simulink model "Reaction_wheel_forse_earth_sensor"  (R2020b)
settings: Solver=VariableStepAuto  StartTime=0.0  StopTime=10.0  RelTol=1e-3
undefined symbols (not defined in the file or in its folder): A, A_star, B, J, Kt, Kw, lw, phi_max, rad, Rm, s, theta_max
libraries: aerolibconvert2 x2, simulink x2, pid_lib x1
settings Model: Creator=jason  LastModifiedBy=jason

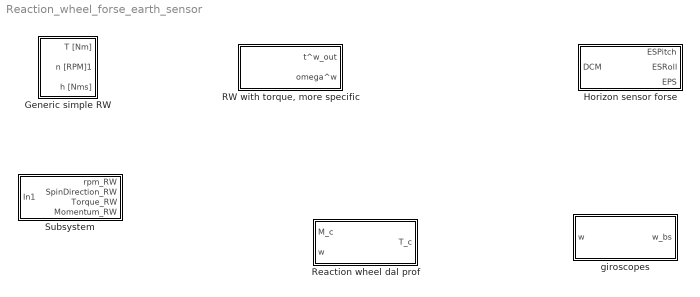
== system Reaction_wheel_forse_earth_sensor ==
  Generic simple RW : Subsystem
  Horizon sensor forse : Subsystem
  "RW with torque, more specific" : Subsystem
  Reaction wheel dal prof : Subsystem
  Subsystem : Subsystem
  giroscopes : Subsystem

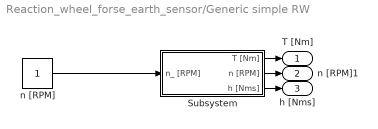
== system Reaction_wheel_forse_earth_sensor/Generic simple RW ==
  Subsystem : Subsystem
  n [RPM] : Constant
  T [Nm] : Outport
  n [RPM]1 : Outport  Port=2
  h [Nms] : Outport  Port=3
  wires:
  Subsystem/2(n [RPM]) -> n [RPM]1/1
  n [RPM]/1 -> Subsystem/1(n_ [RPM])
  Subsystem/1(T [Nm]) -> T [Nm]/1
  Subsystem/3(h [Nms]) -> h [Nms]/1

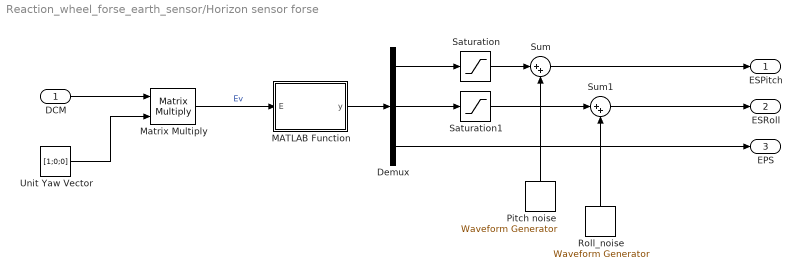
== system Reaction_wheel_forse_earth_sensor/Horizon sensor forse ==
  DCM : Inport
  Demux : Demux  Outputs=3
  MATLAB Function : MATLAB Function  TreatAsAtomicUnit=on
  Matrix Multiply : Product  Multiplication=Matrix(*)
  Pitch noise : simulink/Sources/Waveform Generator  OutMin=[]  OutMax=[]  OutDataTypeStr=double  SelectedSignal=1  BlockNames=MultiportSwitch_e3df3653d217406  SampleTime=0.1
  Roll_noise : simulink/Sources/Waveform Generator  OutMin=[]  OutMax=[]  OutDataTypeStr=double  SelectedSignal=1  BlockNames=MultiportSwitch_e3df3653d217406  SampleTime=0.1
  Saturation : Saturate  UpperLimit=theta_max  LowerLimit=-theta_max
  Saturation1 : Saturate  UpperLimit=phi_max  LowerLimit=-phi_max
  Sum : Sum  Inputs=|++
  Sum1 : Sum  Inputs=|++
  Unit Yaw Vector : Constant  Value=[1;0;0]
  ESPitch : Outport
  ESRoll : Outport  Port=2
  EPS : Outport  Port=3
  wires:
  DCM/1 -> Matrix Multiply/1
  Unit Yaw Vector/1 -> Matrix Multiply/2
  Matrix Multiply/1 -> MATLAB Function/1(E)  "Ev"
  MATLAB Function/1(y) -> Demux/1
  Demux/2 -> Saturation1/1
  Demux/1 -> Saturation/1
  Demux/3 -> EPS/1
  Saturation/1 -> Sum/1
  Saturation1/1 -> Sum1/1
  Sum1/1 -> ESRoll/1
  Sum/1 -> ESPitch/1
  Roll_noise/1 -> Sum1/2
  Pitch noise/1 -> Sum/2

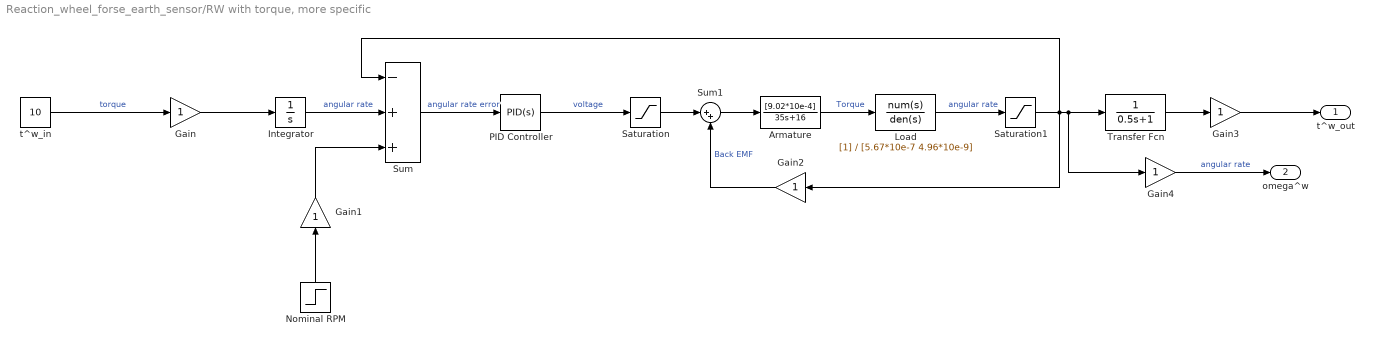
== system Reaction_wheel_forse_earth_sensor/RW with torque, more specific ==
  Armature : TransferFcn  Numerator=[9.02*10e-4]  Denominator=[35 16]  ContinuousStateAttributes='Armature'
  Gain{,1..4} (5 alike) : Gain
  Integrator : Integrator
  Load : TransferFcn  Denominator=[5.67*10e-7 4.96*10e-9]
  Nominal RPM : Step  Time=100  Before=18400  After=36800  SampleTime=0
  PID Controller : pid_lib/PID Controller  Controller=PID  Form=Parallel  TimeDomain=Continuous-time  UseExternalTs=off  SampleTime=-1  IntegratorMethod=Forward Euler  FilterMethod=Forward Euler  ControllerParametersSource=internal  P=9.7  I=0.666  D=0.4  UseFilter=on  N=100  TunerSelectOption=Transfer Function Based (PID Tuner App)  InitialConditionSource=internal  InitialConditionForIntegrator=0  InitialConditionForFilter=0  DifferentiatorICPrevScaledInput=0  ExternalReset=none  TrackingMode=off  Kt=1  LimitOutput=off  SatLimitsSource=internal  UpperSaturationLimit=inf  LowerSaturationLimit=-inf  LinearizeAsGain=on  AntiWindupMode=none  Kb=1  POutMin=[]  POutMax=[]  IOutMin=[]  IOutMax=[]  DOutMin=[]  DOutMax=[]  NOutMin=[]  NOutMax=[]  SumOutMin=[]  SumOutMax=[]  SaturationOutMin=[]  SaturationOutMax=[]  PParamMin=[]  PParamMax=[]  IParamMin=[]  IParamMax=[]  DParamMin=[]  DParamMax=[]  NParamMin=[]  NParamMax=[]  KbParamMin=[]  KbParamMax=[]  KtParamMin=[]  KtParamMax=[]  KbOutMin=[]  KbOutMax=[]  KtOutMin=[]  KtOutMax=[]  IntegratorOutMin=[]  IntegratorOutMax=[]  FilterOutMin=[]  FilterOutMax=[]  SumI1OutMin=[]  SumI1OutMax=[]  SumI2OutMin=[]  SumI2OutMax=[]  SumI3OutMin=[]  SumI3OutMax=[]  SumI4OutMin=[]  SumI4OutMax=[]  SumDOutMin=[]  SumDOutMax=[]  DifferentiatorOutMin=[]  DifferentiatorOutMax=[]  FilterDiffOutCoefMin=[]  FilterDiffOutCoefMax=[]  ReciprocalOutMin=[]  ReciprocalOutMax=[]  SumDenOutMin=[]  SumDenOutMax=[]  SumNumOutMin=[]  SumNumOutMax=[]  DivideOutMin=[]  DivideOutMax=[]  UdiffTsProdOutMin=[]  UdiffTsProdOutMax=[]  NTsProdOutMin=[]  NTsProdOutMax=[]  UintegralTsProdOutMin=[]  UintegralTsProdOutMax=[]  UngainTsProdOutMin=[]  UngainTsProdOutMax=[]  IntegratorContinuousStateAttributes=''  IntegratorStateMustResolveToSignalObject=off  IntegratorRTWStateStorageClass=Auto  FilterContinuousStateAttributes=''  FilterStateMustResolveToSignalObject=off  FilterRTWStateStorageClass=Auto  ParallelPVariant=InternalParameters  IdealPVariant=Disabled  IVariant=InternalParameters  DVariant=InternalParameters  IntegratorVariant=Continuous  SatVariant=Disabled  AWVariant=Passthrough  PCopyVariant=Disabled  TRVariant=Disabled  FdbkBlocksVariant=Forward  IdealPFdbkVariant=Disabled  SatFdbkVariant=Disabled  DerivativeFilterVariant=ContFilter  NVariant=InternalParameters  NCopyVariant=Disabled  FilterICVariant=InternalICsFilter  IntegratorICVariant=InternalICs  ExternalResetVariant=Disabled  TRSumVariant=Passthrough  SumFdbkVariant=Disabled  SumVariant=Sum_PID  TsampFilterVariant=InternalTs  TsampNgainVariant=Passthrough  TsampIntegralVariant=Passthrough  ExternalSaturationOutDataTypeStr=Inherit: Same as second input
  Saturation : Saturate
  Saturation1 : Saturate
  Sum : Sum  Inputs=-++
  Sum1 : Sum  Inputs=|++
  Transfer Fcn : TransferFcn  Denominator=[0.5 1]
  t^w_in : Constant  Value=10
  t^w_out : Outport
  omega^w : Outport  Port=2
  wires:
  Sum1/1 -> Armature/1
  Saturation/1 -> Sum1/1
  PID Controller/1 -> Saturation/1  "voltage"
  Sum/1 -> PID Controller/1  "angular rate error"
  Gain1/1 -> Sum/3
  Integrator/1 -> Sum/2  "angular rate"
  Gain/1 -> Integrator/1
  t^w_in/1 -> Gain/1  "torque"
  Armature/1 -> Load/1  "Torque"
  Load/1 -> Saturation1/1  "angular rate"
  Saturation1/1 -> Gain4/1, Transfer Fcn/1, Sum/1, Gain2/1
  Gain2/1 -> Sum1/2  "Back EMF"
  Transfer Fcn/1 -> Gain3/1
  Gain3/1 -> t^w_out/1
  Gain4/1 -> omega^w/1  "angular rate"
  Nominal RPM/1 -> Gain1/1

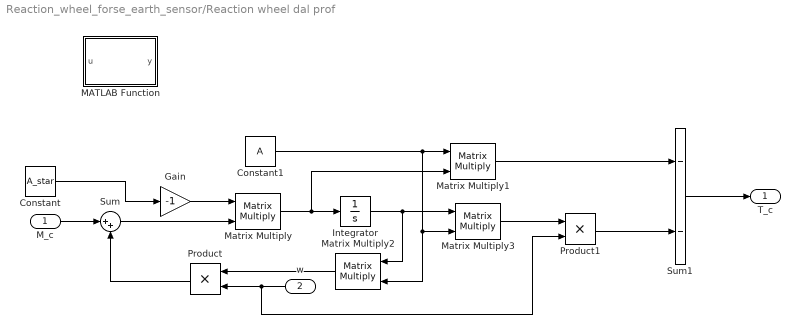
== system Reaction_wheel_forse_earth_sensor/Reaction wheel dal prof ==
  M_c : Inport
  w : Inport  Port=2
  Constant : Constant  Value=A_star
  Constant1 : Constant  Value=A
  Gain : Gain  Gain=-1
  Integrator : Integrator
  MATLAB Function : MATLAB Function  TreatAsAtomicUnit=on
  Matrix Multiply{,1..3} (4 alike) : Product  Multiplication=Matrix(*)
  Product : Product
  Product1 : Product
  Sum : Sum  Inputs=|++
  Sum1 : Sum  Inputs=--
  T_c : Outport
  wires:
  M_c/1 -> Sum/1
  Sum/1 -> Matrix Multiply/2
  Gain/1 -> Matrix Multiply/1
  Constant/1 -> Gain/1
  Matrix Multiply/1 -> Matrix Multiply1/2, Integrator/1
  Integrator/1 -> Matrix Multiply2/1, Matrix Multiply3/1
  Constant1/1 -> Matrix Multiply2/2, Matrix Multiply3/2, Matrix Multiply1/1
  Matrix Multiply1/1 -> Sum1/1
  Sum1/1 -> T_c/1
  w/1 -> Product1/2, Product/2
  Product/1 -> Sum/2
  Matrix Multiply2/1 -> Product/1
  Product1/1 -> Sum1/2
  Matrix Multiply3/1 -> Product1/1

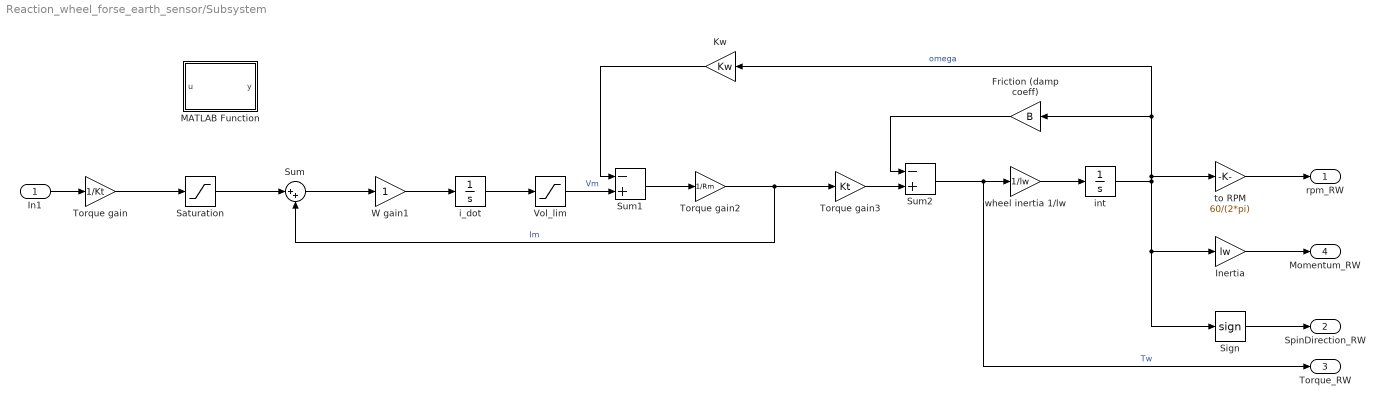
== system Reaction_wheel_forse_earth_sensor/Subsystem ==
  In1 : Inport
  Friction (damp coeff) : Gain  Gain=B
  Inertia : Gain  Gain=lw
  Kw : Gain  Gain=Kw
  MATLAB Function : MATLAB Function  TreatAsAtomicUnit=on
  Saturation : Saturate
  Sign : Signum
  Sum : Sum  Inputs=|++
  Sum1 : Sum  Inputs=-+
  Sum2 : Sum  Inputs=-+
  Torque gain : Gain  Gain=1/Kt
  Torque gain2 : Gain  Gain=1/Rm
  Torque gain3 : Gain  Gain=Kt
  Vol_lim : Saturate
  W gain1 : Gain
  i_dot : Integrator  InitialCondition=[0;0;0]
  int : Integrator  InitialCondition=[0;0;0]
  to RPM : Gain  Gain=60/(2*pi)
  wheel inertia 1/lw : Gain  Gain=1/lw
  rpm_RW : Outport
  SpinDirection_RW : Outport  Port=2
  Torque_RW : Outport  Port=3
  Momentum_RW : Outport  Port=4
  wires:
  In1/1 -> Torque gain/1
  Torque gain/1 -> Saturation/1
  Saturation/1 -> Sum/1
  Sum/1 -> W gain1/1
  W gain1/1 -> i_dot/1
  i_dot/1 -> Vol_lim/1
  Vol_lim/1 -> Sum1/2  "Vm"
  Torque gain2/1 -> Sum/2, Torque gain3/1  "Im"
  Sum1/1 -> Torque gain2/1
  Torque gain3/1 -> Sum2/2
  Friction (damp coeff)/1 -> Sum2/1
  Kw/1 -> Sum1/1
  wheel inertia 1/lw/1 -> int/1
  Sum2/1 -> Torque_RW/1, wheel inertia 1/lw/1  "Tw"
  int/1 -> Kw/1, Friction (damp coeff)/1, to RPM/1, Sign/1, Inertia/1  "omega"
  Sign/1 -> SpinDirection_RW/1
  to RPM/1 -> rpm_RW/1
  Inertia/1 -> Momentum_RW/1

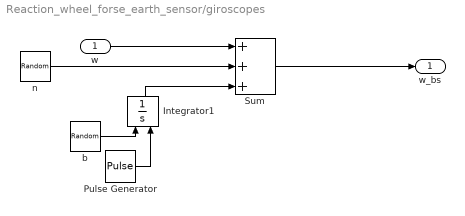
== system Reaction_wheel_forse_earth_sensor/giroscopes ==
  w : Inport
  Integrator1 : Integrator  InitialConditionSource=external
  Pulse Generator : DiscretePulseGenerator  PulseType=Time based  Period=10  PulseWidth=5
  Sum : Sum  Inputs=+++
  b : RandomNumber  SampleTime=0.1
  n : RandomNumber  SampleTime=0.1
  w_bs : Outport
  wires:
  Sum/1 -> w_bs/1
  w/1 -> Sum/1
  n/1 -> Sum/2
  Integrator1/1 -> Sum/3
  Pulse Generator/1 -> Integrator1/2
  b/1 -> Integrator1/1

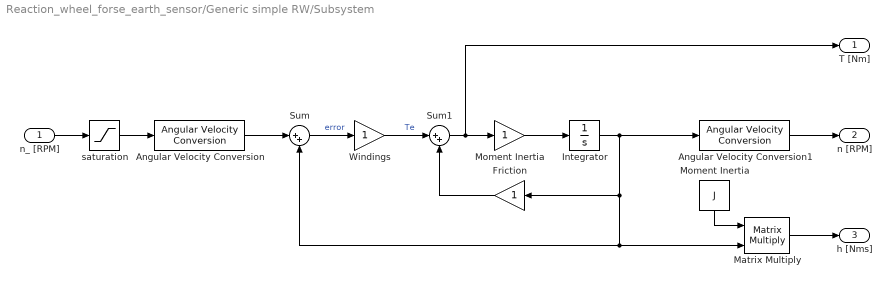
== system Reaction_wheel_forse_earth_sensor/Generic simple RW/Subsystem ==
  n_ [RPM] : Inport
  Angular Velocity Conversion : aerolibconvert2/Angular Velocity Conversion  IU=rpm  OU=rad/s
  Angular Velocity Conversion1 : aerolibconvert2/Angular Velocity Conversion  IU=rad/s  OU=rpm
  Friction : Gain
  Integrator : Integrator
  Matrix Multiply : Product  Multiplication=Matrix(*)
  Moment Inertia : Gain
  "Moment Inertia " : Constant  Value=J
  Sum : Sum  Inputs=|++
  Sum1 : Sum  Inputs=|++
  Windings : Gain
  saturation : Saturate  UpperLimit=10
  T [Nm] : Outport
  n [RPM] : Outport  Port=2
  h [Nms] : Outport  Port=3
  wires:
  n_ [RPM]/1 -> saturation/1
  saturation/1 -> Angular Velocity Conversion/1
  Angular Velocity Conversion/1 -> Sum/1
  Sum/1 -> Windings/1  "error"
  Windings/1 -> Sum1/1  "Te"
  Sum1/1 -> T [Nm]/1, Moment Inertia/1
  Moment Inertia/1 -> Integrator/1
  Integrator/1 -> Angular Velocity Conversion1/1, Sum/2, Matrix Multiply/2, Friction/1
  Friction/1 -> Sum1/2
  Matrix Multiply/1 -> h [Nms]/1
  "Moment Inertia "/1 -> Matrix Multiply/1
  Angular Velocity Conversion1/1 -> n [RPM]/1

== matlab function Reaction_wheel_forse_earth_sensor/Subsystem/MATLAB Function ==
  data: u input; y output
function y = fun_per_RW(u)

Kw = 0.001; % back EMF
Kt = 0.5; % torque gain
K = 1; % wheel gain
B = 0.000102; % friction torque
lw = 0.035; % wheel inertia
Rm = 1; % Rotor Resistance

== matlab function Reaction_wheel_forse_earth_sensor/Reaction wheel dal prof/MATLAB Function ==
  data: u input; y output
function y = fcn(u)
e = 1/sqrt(3);
A = [1 0 0 e;
    0 1 0 e;
    0 0 1 e];
a = 5/6;
b = -1/6;
c = 1/(2*sqrt(3));

A_star = [a b b;
    b a b;
    b b a;
    c c c];
y = [A A_star];

== matlab function Reaction_wheel_forse_earth_sensor/Horizon sensor forse/MATLAB Function ==
  data: E input; y output
function y = fcn(E)

Evx = E(1);
Evy = E(2);
Evz = E(3);
ee = [Evx Evy];
theta = atan(-(Evy)/(Evx));
phi = atan(Evz/(norm(ee)));
EPS = Evz;



y = [theta phi EPS];
